simulink model "CEN598_HW2"  (R2015b)
settings: Solver=FixedStepDiscrete  SolverMode=SingleTasking  StartTime=0.0  StopTime=2.5e-6  RelTol=1e-3
libraries: shlslibv1 x212
(part 2 of 2)

== system CEN598_HW2/Interleaved MAC PE11/MAC PE ==
  x_i : Inport
  a_ij : Inport  Port=2
  FP Add : shlslibv1/Floating Point/FP Add  syn_exp_wl=11  syn_frac_wl=52  syn_opt_ports=off  syn_add_opr=add  synBlockType=custom  synLatency=9
  FP Constant : shlslibv1/Floating Point/FP Constant  syn_constant_val=1  syn_exp_wl=11  syn_frac_wl=52  syn_cst_st=1/284.04e6  synBlockType=custom  synLatency=0
  FP Mult : shlslibv1/Floating Point/FP Mult  syn_exp_wl=11  syn_frac_wl=52  syn_opt_ports=off  synBlockType=custom  synLatency=3  syn_opt_tar=Default  syn_fracmult_pipe=1
  Terminator : Terminator
  y_1 : Outport
  wires:
  x_i/1 -> FP Mult/1
  a_ij/1 -> FP Mult/2
  FP Mult/1 -> FP Add/2
  FP Mult/2 -> FP Add/3
  FP Add/1 -> FP Add/1, y_1/1
  FP Add/2 -> Terminator/1
  FP Constant/1 -> FP Mult/3

== system CEN598_HW2/Interleaved MAC PE12/MAC PE ==
  x_i : Inport
  a_ij : Inport  Port=2
  FP Add : shlslibv1/Floating Point/FP Add  syn_exp_wl=11  syn_frac_wl=52  syn_opt_ports=off  syn_add_opr=add  synBlockType=custom  synLatency=9
  FP Constant : shlslibv1/Floating Point/FP Constant  syn_constant_val=1  syn_exp_wl=11  syn_frac_wl=52  syn_cst_st=1/284.04e6  synBlockType=custom  synLatency=0
  FP Mult : shlslibv1/Floating Point/FP Mult  syn_exp_wl=11  syn_frac_wl=52  syn_opt_ports=off  synBlockType=custom  synLatency=3  syn_opt_tar=Default  syn_fracmult_pipe=1
  Terminator : Terminator
  y_1 : Outport
  wires:
  x_i/1 -> FP Mult/1
  a_ij/1 -> FP Mult/2
  FP Mult/1 -> FP Add/2
  FP Mult/2 -> FP Add/3
  FP Add/1 -> FP Add/1, y_1/1
  FP Add/2 -> Terminator/1
  FP Constant/1 -> FP Mult/3

== system CEN598_HW2/Interleaved MAC PE13/MAC PE ==
  x_i : Inport
  a_ij : Inport  Port=2
  FP Add : shlslibv1/Floating Point/FP Add  syn_exp_wl=11  syn_frac_wl=52  syn_opt_ports=off  syn_add_opr=add  synBlockType=custom  synLatency=9
  FP Constant : shlslibv1/Floating Point/FP Constant  syn_constant_val=1  syn_exp_wl=11  syn_frac_wl=52  syn_cst_st=1/284.04e6  synBlockType=custom  synLatency=0
  FP Mult : shlslibv1/Floating Point/FP Mult  syn_exp_wl=11  syn_frac_wl=52  syn_opt_ports=off  synBlockType=custom  synLatency=3  syn_opt_tar=Default  syn_fracmult_pipe=1
  Terminator : Terminator
  y_1 : Outport
  wires:
  x_i/1 -> FP Mult/1
  a_ij/1 -> FP Mult/2
  FP Mult/1 -> FP Add/2
  FP Mult/2 -> FP Add/3
  FP Add/1 -> FP Add/1, y_1/1
  FP Add/2 -> Terminator/1
  FP Constant/1 -> FP Mult/3

== system CEN598_HW2/Interleaved MAC PE14/MAC PE ==
  x_i : Inport
  a_ij : Inport  Port=2
  FP Add : shlslibv1/Floating Point/FP Add  syn_exp_wl=11  syn_frac_wl=52  syn_opt_ports=off  syn_add_opr=add  synBlockType=custom  synLatency=9
  FP Constant : shlslibv1/Floating Point/FP Constant  syn_constant_val=1  syn_exp_wl=11  syn_frac_wl=52  syn_cst_st=1/284.04e6  synBlockType=custom  synLatency=0
  FP Mult : shlslibv1/Floating Point/FP Mult  syn_exp_wl=11  syn_frac_wl=52  syn_opt_ports=off  synBlockType=custom  synLatency=3  syn_opt_tar=Default  syn_fracmult_pipe=1
  Terminator : Terminator
  y_1 : Outport
  wires:
  x_i/1 -> FP Mult/1
  a_ij/1 -> FP Mult/2
  FP Mult/1 -> FP Add/2
  FP Mult/2 -> FP Add/3
  FP Add/1 -> FP Add/1, y_1/1
  FP Add/2 -> Terminator/1
  FP Constant/1 -> FP Mult/3

== system CEN598_HW2/Interleaved MAC PE15/MAC PE ==
  x_i : Inport
  a_ij : Inport  Port=2
  FP Add : shlslibv1/Floating Point/FP Add  syn_exp_wl=11  syn_frac_wl=52  syn_opt_ports=off  syn_add_opr=add  synBlockType=custom  synLatency=9
  FP Constant : shlslibv1/Floating Point/FP Constant  syn_constant_val=1  syn_exp_wl=11  syn_frac_wl=52  syn_cst_st=1/284.04e6  synBlockType=custom  synLatency=0
  FP Mult : shlslibv1/Floating Point/FP Mult  syn_exp_wl=11  syn_frac_wl=52  syn_opt_ports=off  synBlockType=custom  synLatency=3  syn_opt_tar=Default  syn_fracmult_pipe=1
  Terminator : Terminator
  y_1 : Outport
  wires:
  x_i/1 -> FP Mult/1
  a_ij/1 -> FP Mult/2
  FP Mult/1 -> FP Add/2
  FP Mult/2 -> FP Add/3
  FP Add/1 -> FP Add/1, y_1/1
  FP Add/2 -> Terminator/1
  FP Constant/1 -> FP Mult/3

== system CEN598_HW2/Interleaved MAC PE2/MAC PE ==
  x_i : Inport
  a_ij : Inport  Port=2
  FP Add : shlslibv1/Floating Point/FP Add  syn_exp_wl=11  syn_frac_wl=52  syn_opt_ports=off  syn_add_opr=add  synBlockType=custom  synLatency=9
  FP Constant : shlslibv1/Floating Point/FP Constant  syn_constant_val=1  syn_exp_wl=11  syn_frac_wl=52  syn_cst_st=1/284.04e6  synBlockType=custom  synLatency=0
  FP Mult : shlslibv1/Floating Point/FP Mult  syn_exp_wl=11  syn_frac_wl=52  syn_opt_ports=off  synBlockType=custom  synLatency=3  syn_opt_tar=Default  syn_fracmult_pipe=1
  Terminator : Terminator
  y_1 : Outport
  wires:
  x_i/1 -> FP Mult/1
  a_ij/1 -> FP Mult/2
  FP Mult/1 -> FP Add/2
  FP Mult/2 -> FP Add/3
  FP Add/1 -> FP Add/1, y_1/1
  FP Add/2 -> Terminator/1
  FP Constant/1 -> FP Mult/3

== system CEN598_HW2/Interleaved MAC PE3/MAC PE ==
  x_i : Inport
  a_ij : Inport  Port=2
  FP Add : shlslibv1/Floating Point/FP Add  syn_exp_wl=11  syn_frac_wl=52  syn_opt_ports=off  syn_add_opr=add  synBlockType=custom  synLatency=9
  FP Constant : shlslibv1/Floating Point/FP Constant  syn_constant_val=1  syn_exp_wl=11  syn_frac_wl=52  syn_cst_st=1/284.04e6  synBlockType=custom  synLatency=0
  FP Mult : shlslibv1/Floating Point/FP Mult  syn_exp_wl=11  syn_frac_wl=52  syn_opt_ports=off  synBlockType=custom  synLatency=3  syn_opt_tar=Default  syn_fracmult_pipe=1
  Terminator : Terminator
  y_1 : Outport
  wires:
  x_i/1 -> FP Mult/1
  a_ij/1 -> FP Mult/2
  FP Mult/1 -> FP Add/2
  FP Mult/2 -> FP Add/3
  FP Add/1 -> FP Add/1, y_1/1
  FP Add/2 -> Terminator/1
  FP Constant/1 -> FP Mult/3

== system CEN598_HW2/Interleaved MAC PE4/MAC PE ==
  x_i : Inport
  a_ij : Inport  Port=2
  FP Add : shlslibv1/Floating Point/FP Add  syn_exp_wl=11  syn_frac_wl=52  syn_opt_ports=off  syn_add_opr=add  synBlockType=custom  synLatency=9
  FP Constant : shlslibv1/Floating Point/FP Constant  syn_constant_val=1  syn_exp_wl=11  syn_frac_wl=52  syn_cst_st=1/284.04e6  synBlockType=custom  synLatency=0
  FP Mult : shlslibv1/Floating Point/FP Mult  syn_exp_wl=11  syn_frac_wl=52  syn_opt_ports=off  synBlockType=custom  synLatency=3  syn_opt_tar=Default  syn_fracmult_pipe=1
  Terminator : Terminator
  y_1 : Outport
  wires:
  x_i/1 -> FP Mult/1
  a_ij/1 -> FP Mult/2
  FP Mult/1 -> FP Add/2
  FP Mult/2 -> FP Add/3
  FP Add/1 -> FP Add/1, y_1/1
  FP Add/2 -> Terminator/1
  FP Constant/1 -> FP Mult/3

== system CEN598_HW2/Interleaved MAC PE5/MAC PE ==
  x_i : Inport
  a_ij : Inport  Port=2
  FP Add : shlslibv1/Floating Point/FP Add  syn_exp_wl=11  syn_frac_wl=52  syn_opt_ports=off  syn_add_opr=add  synBlockType=custom  synLatency=9
  FP Constant : shlslibv1/Floating Point/FP Constant  syn_constant_val=1  syn_exp_wl=11  syn_frac_wl=52  syn_cst_st=1/284.04e6  synBlockType=custom  synLatency=0
  FP Mult : shlslibv1/Floating Point/FP Mult  syn_exp_wl=11  syn_frac_wl=52  syn_opt_ports=off  synBlockType=custom  synLatency=3  syn_opt_tar=Default  syn_fracmult_pipe=1
  Terminator : Terminator
  y_1 : Outport
  wires:
  x_i/1 -> FP Mult/1
  a_ij/1 -> FP Mult/2
  FP Mult/1 -> FP Add/2
  FP Mult/2 -> FP Add/3
  FP Add/1 -> FP Add/1, y_1/1
  FP Add/2 -> Terminator/1
  FP Constant/1 -> FP Mult/3

== system CEN598_HW2/Interleaved MAC PE6/MAC PE ==
  x_i : Inport
  a_ij : Inport  Port=2
  FP Add : shlslibv1/Floating Point/FP Add  syn_exp_wl=11  syn_frac_wl=52  syn_opt_ports=off  syn_add_opr=add  synBlockType=custom  synLatency=9
  FP Constant : shlslibv1/Floating Point/FP Constant  syn_constant_val=1  syn_exp_wl=11  syn_frac_wl=52  syn_cst_st=1/284.04e6  synBlockType=custom  synLatency=0
  FP Mult : shlslibv1/Floating Point/FP Mult  syn_exp_wl=11  syn_frac_wl=52  syn_opt_ports=off  synBlockType=custom  synLatency=3  syn_opt_tar=Default  syn_fracmult_pipe=1
  Terminator : Terminator
  y_1 : Outport
  wires:
  x_i/1 -> FP Mult/1
  a_ij/1 -> FP Mult/2
  FP Mult/1 -> FP Add/2
  FP Mult/2 -> FP Add/3
  FP Add/1 -> FP Add/1, y_1/1
  FP Add/2 -> Terminator/1
  FP Constant/1 -> FP Mult/3

== system CEN598_HW2/Interleaved MAC PE7/MAC PE ==
  x_i : Inport
  a_ij : Inport  Port=2
  FP Add : shlslibv1/Floating Point/FP Add  syn_exp_wl=11  syn_frac_wl=52  syn_opt_ports=off  syn_add_opr=add  synBlockType=custom  synLatency=9
  FP Constant : shlslibv1/Floating Point/FP Constant  syn_constant_val=1  syn_exp_wl=11  syn_frac_wl=52  syn_cst_st=1/284.04e6  synBlockType=custom  synLatency=0
  FP Mult : shlslibv1/Floating Point/FP Mult  syn_exp_wl=11  syn_frac_wl=52  syn_opt_ports=off  synBlockType=custom  synLatency=3  syn_opt_tar=Default  syn_fracmult_pipe=1
  Terminator : Terminator
  y_1 : Outport
  wires:
  x_i/1 -> FP Mult/1
  a_ij/1 -> FP Mult/2
  FP Mult/1 -> FP Add/2
  FP Mult/2 -> FP Add/3
  FP Add/1 -> FP Add/1, y_1/1
  FP Add/2 -> Terminator/1
  FP Constant/1 -> FP Mult/3

== system CEN598_HW2/Interleaved MAC PE8/MAC PE ==
  x_i : Inport
  a_ij : Inport  Port=2
  FP Add : shlslibv1/Floating Point/FP Add  syn_exp_wl=11  syn_frac_wl=52  syn_opt_ports=off  syn_add_opr=add  synBlockType=custom  synLatency=9
  FP Constant : shlslibv1/Floating Point/FP Constant  syn_constant_val=1  syn_exp_wl=11  syn_frac_wl=52  syn_cst_st=1/284.04e6  synBlockType=custom  synLatency=0
  FP Mult : shlslibv1/Floating Point/FP Mult  syn_exp_wl=11  syn_frac_wl=52  syn_opt_ports=off  synBlockType=custom  synLatency=3  syn_opt_tar=Default  syn_fracmult_pipe=1
  Terminator : Terminator
  y_1 : Outport
  wires:
  x_i/1 -> FP Mult/1
  a_ij/1 -> FP Mult/2
  FP Mult/1 -> FP Add/2
  FP Mult/2 -> FP Add/3
  FP Add/1 -> FP Add/1, y_1/1
  FP Add/2 -> Terminator/1
  FP Constant/1 -> FP Mult/3

== system CEN598_HW2/Interleaved MAC PE9/MAC PE ==
  x_i : Inport
  a_ij : Inport  Port=2
  FP Add : shlslibv1/Floating Point/FP Add  syn_exp_wl=11  syn_frac_wl=52  syn_opt_ports=off  syn_add_opr=add  synBlockType=custom  synLatency=9
  FP Constant : shlslibv1/Floating Point/FP Constant  syn_constant_val=1  syn_exp_wl=11  syn_frac_wl=52  syn_cst_st=1/284.04e6  synBlockType=custom  synLatency=0
  FP Mult : shlslibv1/Floating Point/FP Mult  syn_exp_wl=11  syn_frac_wl=52  syn_opt_ports=off  synBlockType=custom  synLatency=3  syn_opt_tar=Default  syn_fracmult_pipe=1
  Terminator : Terminator
  y_1 : Outport
  wires:
  x_i/1 -> FP Mult/1
  a_ij/1 -> FP Mult/2
  FP Mult/1 -> FP Add/2
  FP Mult/2 -> FP Add/3
  FP Add/1 -> FP Add/1, y_1/1
  FP Add/2 -> Terminator/1
  FP Constant/1 -> FP Mult/3
